simulink model "fourorder"  (R2023b)
settings: Solver=FixedStepAuto  StartTime=0.0  StopTime=100  FixedStep=0.001  RelTol=1e-3
values from neighbouring files (symbols this model uses):
  A = [-0.607110322581 0.050179746608 0 0 1 0 0 0.150121075269 -0.118469799623 0.253333333333 0 -1 ... (49 elements, 7x7)]    [data.mat]    (also in string1.m = [-(c1+cr)/J1 c1/J1 0 0 -k1/J1 0 0)
  AA = [-0.607110322581 0.050179746608 0 0 1 0 0 -1 0.150121075269 -0.118469799623 0.253333333333 0 ... (64 elements, 8x8)]    [data.mat]
  B = [0.0010752688172 0 0 0 0 0 0]    [data.mat]
  B2 = [0 0 0 -0.00211877963378 0 0 0 0.0010752688172 0 0 0 0 ... (14 elements, 7x2)]    [data.mat]    (also in demo_pid.m = -J \ [0; 1]; string1.m = [0 1/J1;0 0;0 0;-1/J4 0 ;0 0;0 0;0 0])
  BB = [0.0010752688172 0 0 0 0 0 0 0]    [data.mat]
  Bw = [0 0 0 -0.00211877963378 0 0 0 0]    [data.mat]
  C = [1 0 0 0 0 0 0]    [data.mat]    (also in string1.m = [1 0 0 0 0 0 0)
  C_3 = [1 0 0 0 0 0 0 0 0 0 0 1 ... (24 elements, 3x8)]    [data.mat]
  C_37 = [1 0 0 0 0 0 0 0 0 0 0 1 ... (21 elements, 3x7)]    [data.mat]
  G = [12.2186235804 178.38475641 -301.660194136 -80.857185539 -52.8926654988 -580.80827196 633.197555561]    [data.mat]
libraries: slpidlib x2, fuzblock x1
settings Model: Creator=ASUS  LastModifiedBy=86188
settings SolverCC: AlgebraicLoopSolver=TrustRegion
settings DebuggingCC: UnconnectedInputMsg=warning  UnconnectedOutputMsg=warning  UnconnectedLineMsg=warning
settings ModelReferenceCC: EnableRefExpFcnMdlSchedulingChecks=on
settings RTWCC: DLArmComputeVersion=19.05

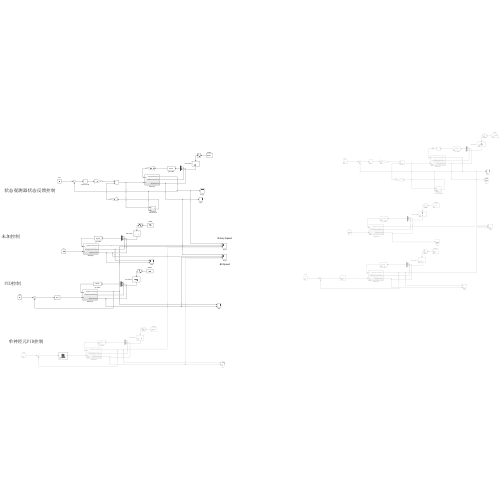
[thumbnail: Simulink's stored preview of the top-level diagram]
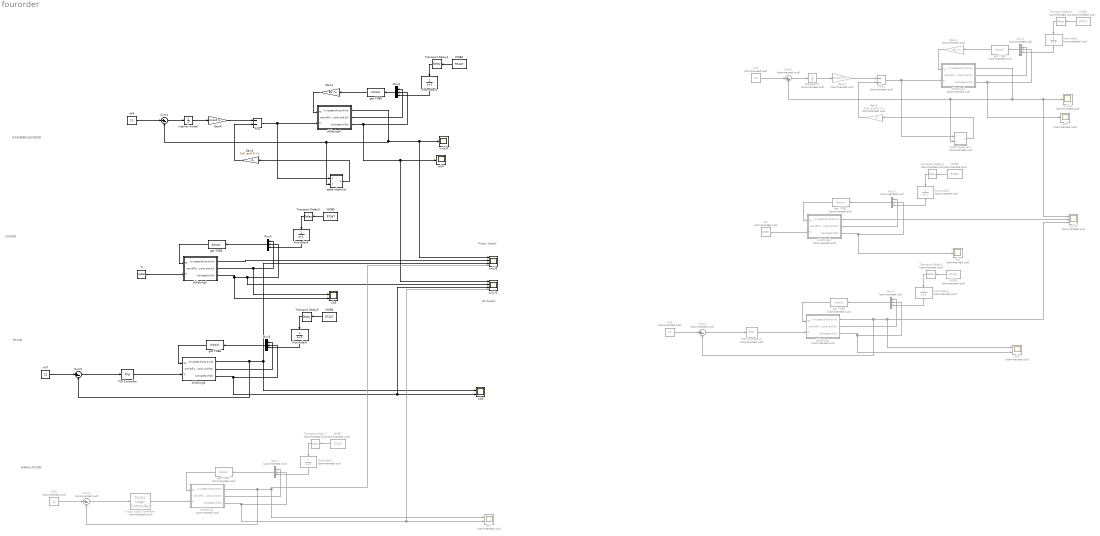
== system fourorder ==
  note: Rotary Speed
  note: 状态观测器状态反馈控制
  note: 未加控制
  note: PID控制
  note: Bit Speed
  note: 单神经元PID控制
  Fuzzy Logic Controller : fuzblock/Fuzzy Logic  Controller  Commented=on  FIS='drill.fis'  OutputSampleNumber=101  DataType=double  FuzzifiedInputs=off  RuleFiringStrengths=off  RuleOutputs=off  AggregatedOutputs=off  SimulateUsing=Interpreted execution  OutOfRangeInputValueMessage=warning  NoRuleFiredMessage=warning  EmptyOutputFuzzySetMessage=warning
  Gain1 : Gain  Commented=on  Gain=Bw  Multiplication=Matrix(K*u)
  Gain2 : Gain  Commented=on  Gain=Ks(1:end-1)  Multiplication=Matrix(K*u)
  Gain3 : Gain  Commented=on  Gain=Ks(end)  Multiplication=Matrix(K*u)
  Gain4 : Gain  Gain=Bw  Multiplication=Matrix(K*u)
  Gain5 : Gain  Gain=Ks(1:end-1)  Multiplication=Matrix(K*u)
  Gain6 : Gain  Gain=Ks(end)  Multiplication=Matrix(K*u)
  Integrator1 : Integrator  Commented=on
  Mux{1..3,7} (4 alike) : Mux  Commented=on  Inputs=3
  Mux4 : Mux  Inputs=3
  Mux5 : Mux  Inputs=3
  Mux6 : Mux  Inputs=3
  PID Controller : slpidlib/PID Controller  Controller=PI  Form=Parallel  TimeDomain=Continuous-time  UseExternalTs=off  SampleTime=-1  IntegratorMethod=Forward Euler  FilterMethod=Forward Euler  ControllerParametersSource=internal  P=1500  I=300  UseKiTs=off  D=0  N=100  UseFilter=on  TunerSelectOption=Transfer Function Based (PID Tuner App)  InitialConditionSource=internal  InitialConditionForIntegrator=0  InitialConditionForFilter=0  DifferentiatorICPrevScaledInput=0  ExternalReset=none  TrackingMode=off  Kt=1  LimitOutput=off  SatLimitsSource=internal  UpperSaturationLimit=inf  LowerSaturationLimit=-inf  LinearizeAsGain=on  AntiWindupMode=none  Kb=1  LimitIntegrator=off  UpperIntegratorSaturationLimit=inf  LowerIntegratorSaturationLimit=-inf  POutMin=[]  POutMax=[]  IOutMin=[]  IOutMax=[]  DOutMin=[]  DOutMax=[]  NOutMin=[]  NOutMax=[]  SumOutMin=[]  SumOutMax=[]  SaturationOutMin=[]  SaturationOutMax=[]  PParamMin=[]  PParamMax=[]  IParamMin=[]  IParamMax=[]  DParamMin=[]  DParamMax=[]  NParamMin=[]  NParamMax=[]  KbParamMin=[]  KbParamMax=[]  KtParamMin=[]  KtParamMax=[]  KbOutMin=[]  KbOutMax=[]  KtOutMin=[]  KtOutMax=[]  IntegratorOutMin=[]  IntegratorOutMax=[]  FilterOutMin=[]  FilterOutMax=[]  SumI1OutMin=[]  SumI1OutMax=[]  SumI2OutMin=[]  SumI2OutMax=[]  SumI3OutMin=[]  SumI3OutMax=[]  SumI4OutMin=[]  SumI4OutMax=[]  SumDOutMin=[]  SumDOutMax=[]  DifferentiatorOutMin=[]  DifferentiatorOutMax=[]  FilterDiffOutCoefMin=[]  FilterDiffOutCoefMax=[]  ReciprocalOutMin=[]  ReciprocalOutMax=[]  SumDenOutMin=[]  SumDenOutMax=[]  SumNumOutMin=[]  SumNumOutMax=[]  DivideOutMin=[]  DivideOutMax=[]  UdiffTsProdOutMin=[]  UdiffTsProdOutMax=[]  NTsProdOutMin=[]  NTsProdOutMax=[]  UintegralTsProdOutMin=[]  UintegralTsProdOutMax=[]  UngainTsProdOutMin=[]  UngainTsProdOutMax=[]  ClampingZeroOutDataTypeStr=Inherit: Inherit via back propagation  ClampingZeroOutMin=[]  ClampingZeroOutMax=[]  FilterDenConstantOutDataTypeStr=Inherit: Inherit via back propagation  FilterDenConstantOutMin=[]  FilterDenConstantOutMax=[]  PCopyOutDataTypeStr=Inherit: Inherit via back propagation  PCopyOutMin=[]  PCopyOutMax=[]  NCopyOutDataTypeStr=Inherit: Inherit via back propagation  NCopyOutMin=[]  NCopyOutMax=[]  IntegratorContinuousStateAttributes=''  IntegratorStateMustResolveToSignalObject=off  IntegratorRTWStateStorageClass=Auto  FilterContinuousStateAttributes=''  FilterStateMustResolveToSignalObject=off  FilterRTWStateStorageClass=Auto  ParallelPVariant=InternalParameters  IdealPVariant=Disabled  IVariant=InternalParameters  DVariant=Disabled  IntegratorVariant=Continuous  SatVariant=Disabled  AWVariant=Passthrough  PCopyVariant=Disabled  TRVariant=Disabled  FdbkBlocksVariant=Forward  IdealPFdbkVariant=Disabled  SatFdbkVariant=Disabled  DerivativeFilterVariant=Disabled  NVariant=Disabled  NCopyVariant=Disabled_SignalSpec  FilterICVariant=Disabled  IntegratorICVariant=InternalICs  ExternalResetVariant=Disabled  TRSumVariant=Passthrough  SumFdbkVariant=Disabled  SumVariant=Sum_PI  TsampFilterVariant=InternalTs  TsampNgainVariant=Passthrough  TsampIntegralVariant=Disabled_SignalSpec  ExternalSaturationOutDataTypeStr=Inherit: Same as second input
  PID Controller1 : slpidlib/PID Controller  Commented=on  Controller=PI  Form=Parallel  TimeDomain=Continuous-time  UseExternalTs=off  SampleTime=-1  IntegratorMethod=Forward Euler  FilterMethod=Forward Euler  ControllerParametersSource=internal  P=1000  I=100  UseKiTs=off  D=0  N=100  UseFilter=on  TunerSelectOption=Transfer Function Based (PID Tuner App)  InitialConditionSource=internal  InitialConditionForIntegrator=0  InitialConditionForFilter=0  DifferentiatorICPrevScaledInput=0  ExternalReset=none  TrackingMode=off  Kt=1  LimitOutput=off  SatLimitsSource=internal  UpperSaturationLimit=inf  LowerSaturationLimit=-inf  LinearizeAsGain=on  AntiWindupMode=none  Kb=1  LimitIntegrator=off  UpperIntegratorSaturationLimit=inf  LowerIntegratorSaturationLimit=-inf  POutMin=[]  POutMax=[]  IOutMin=[]  IOutMax=[]  DOutMin=[]  DOutMax=[]  NOutMin=[]  NOutMax=[]  SumOutMin=[]  SumOutMax=[]  SaturationOutMin=[]  SaturationOutMax=[]  PParamMin=[]  PParamMax=[]  IParamMin=[]  IParamMax=[]  DParamMin=[]  DParamMax=[]  NParamMin=[]  NParamMax=[]  KbParamMin=[]  KbParamMax=[]  KtParamMin=[]  KtParamMax=[]  KbOutMin=[]  KbOutMax=[]  KtOutMin=[]  KtOutMax=[]  IntegratorOutMin=[]  IntegratorOutMax=[]  FilterOutMin=[]  FilterOutMax=[]  SumI1OutMin=[]  SumI1OutMax=[]  SumI2OutMin=[]  SumI2OutMax=[]  SumI3OutMin=[]  SumI3OutMax=[]  SumI4OutMin=[]  SumI4OutMax=[]  SumDOutMin=[]  SumDOutMax=[]  DifferentiatorOutMin=[]  DifferentiatorOutMax=[]  FilterDiffOutCoefMin=[]  FilterDiffOutCoefMax=[]  ReciprocalOutMin=[]  ReciprocalOutMax=[]  SumDenOutMin=[]  SumDenOutMax=[]  SumNumOutMin=[]  SumNumOutMax=[]  DivideOutMin=[]  DivideOutMax=[]  UdiffTsProdOutMin=[]  UdiffTsProdOutMax=[]  NTsProdOutMin=[]  NTsProdOutMax=[]  UintegralTsProdOutMin=[]  UintegralTsProdOutMax=[]  UngainTsProdOutMin=[]  UngainTsProdOutMax=[]  ClampingZeroOutDataTypeStr=Inherit: Inherit via back propagation  ClampingZeroOutMin=[]  ClampingZeroOutMax=[]  FilterDenConstantOutDataTypeStr=Inherit: Inherit via back propagation  FilterDenConstantOutMin=[]  FilterDenConstantOutMax=[]  PCopyOutDataTypeStr=Inherit: Inherit via back propagation  PCopyOutMin=[]  PCopyOutMax=[]  NCopyOutDataTypeStr=Inherit: Inherit via back propagation  NCopyOutMin=[]  NCopyOutMax=[]  IntegratorContinuousStateAttributes=''  IntegratorStateMustResolveToSignalObject=off  IntegratorRTWStateStorageClass=Auto  FilterContinuousStateAttributes=''  FilterStateMustResolveToSignalObject=off  FilterRTWStateStorageClass=Auto  ParallelPVariant=InternalParameters  IdealPVariant=Disabled  IVariant=InternalParameters  DVariant=Disabled  IntegratorVariant=Continuous  SatVariant=Disabled  AWVariant=Passthrough  PCopyVariant=Disabled  TRVariant=Disabled  FdbkBlocksVariant=Forward  IdealPFdbkVariant=Disabled  SatFdbkVariant=Disabled  DerivativeFilterVariant=Disabled  NVariant=Disabled  NCopyVariant=Disabled_SignalSpec  FilterICVariant=Disabled  IntegratorICVariant=InternalICs  ExternalResetVariant=Disabled  TRSumVariant=Passthrough  SumFdbkVariant=Disabled  SumVariant=Sum_PI  TsampFilterVariant=InternalTs  TsampNgainVariant=Passthrough  TsampIntegralVariant=Disabled_SignalSpec  ExternalSaturationOutDataTypeStr=Inherit: Same as second input
  Plus : Sum  Inputs=--
  Plus1 : Sum  Commented=on  Inputs=--
  Sum1 : Sum  Commented=on  Inputs=|+-
  Sum2 : Sum  Commented=on  Inputs=|+-
  Sum3 : Sum  Commented=on  Inputs=|+-
  Sum4 : Sum  Inputs=|+-
  Sum5 : Sum  Inputs=|+-
  Tr : Constant  Value=10000
  Tr1 : Constant  Commented=on  Value=10000
  Transport Delay{1..3,7} (4 alike) : TransportDelay  Commented=on  DelayTime=50  InitialOutput=100000
  Transport Delay4 : TransportDelay  DelayTime=50  InitialOutput=100000
  Transport Delay5 : TransportDelay  DelayTime=50  InitialOutput=100000
  Transport Delay6 : TransportDelay  DelayTime=50  InitialOutput=100000
  WOB{1..3,7} (4 alike) : Constant  Commented=on  Value=97347
  WOB4 : Constant  Value=97347
  WOB5 : Constant  Value=97347
  WOB6 : Constant  Value=97347
  drillstring1 : Subsystem  Commented=on
  drillstring2 : Subsystem  Commented=on
  drillstring3 : Subsystem  Commented=on
  drillstring4 : Subsystem
  drillstring5 : Subsystem
  drillstring6 : Subsystem
  drillstring7 : Subsystem  Commented=on
  first-order{1..3,7} (4 alike) : TransferFcn  Commented=on  Denominator=[1 1]
  first-order4 : TransferFcn  Denominator=[1 1]
  first-order5 : TransferFcn  Denominator=[1 1]
  first-order6 : TransferFcn  Denominator=[1 1]
  get TOB{1..3,7} (4 alike) : S-Function  Commented=on  FunctionName=bitrock  SFunctionDeploymentMode=off  EnableBusSupport=off
  get TOB4 : S-Function  FunctionName=bitrock  SFunctionDeploymentMode=off  EnableBusSupport=off
  get TOB5 : S-Function  FunctionName=bitrock  SFunctionDeploymentMode=off  EnableBusSupport=off
  get TOB6 : S-Function  FunctionName=bitrock  SFunctionDeploymentMode=off  EnableBusSupport=off
  internal model : Integrator
  r(t)1 : Constant  Commented=on  Value=12
  r(t)2 : Constant  Commented=on  Value=12
  r(t)3 : Constant  Commented=on  Value=12
  r(t)4 : Constant  Value=12
  r(t)7 : Constant  Value=12
  state observer : Subsystem
  state observer1 : Subsystem  Commented=on
  wb1 : Scope  Commented=on
  wb2 : Scope  Commented=on
  wb3 : Scope  Commented=on  NumInputPorts=2
  wb4 : Scope
  wb5 : Scope  NumInputPorts=2
  wb6 : Scope  NumInputPorts=2
  wb7 : Scope  Commented=on  NumInputPorts=2
  wr(y)1 : Scope  Commented=on
  wr(y)2 : Scope  Commented=on  NumInputPorts=3
  wr(y)3 : Scope  NumInputPorts=4
  wr(y)4 : Scope
  wr(y)5 : Scope  NumInputPorts=4
  wires:
  state observer/1(Out1) -> Gain5/1
  first-order4/1 -> Mux4/3
  Transport Delay4/1 -> first-order4/1
  drillstring4/3(wb(speed of bit)) -> wr(y)3/1, wb4/1, Mux4/2
  Mux4/1 -> get TOB4/1
  drillstring4/2(wer(diff of collar and bit)) -> Mux4/1
  drillstring4/1(wr(speed of top drive)) -> Sum4/2, state observer/2(In2), wr(y)5/1, wr(y)4/1
  r(t)4/1 -> Sum4/1
  Sum4/1 -> internal model/1
  WOB4/1 -> Transport Delay4/1
  get TOB4/1 -> Gain4/1
  Plus/1 -> drillstring4/2(Tr), state observer/1(In1)
  Gain5/1 -> Plus/2
  Gain6/1 -> Plus/1
  internal model/1 -> Gain6/1
  Gain4/1 -> drillstring4/1(Tb)
  drillstring5/1(wr(speed of top drive)) -> wr(y)5/2
  WOB5/1 -> Transport Delay5/1
  drillstring5/2(wer(diff of collar and bit)) -> wb5/1, Mux5/1
  first-order5/1 -> Mux5/3
  Mux5/1 -> get TOB5/1
  drillstring5/3(wb(speed of bit)) -> wb5/2, wr(y)3/2, Mux5/2
  get TOB5/1 -> drillstring5/1(Tb)
  Transport Delay5/1 -> first-order5/1
  Tr/1 -> drillstring5/2(Tr)
  Sum5/1 -> PID Controller/1
  drillstring6/2(wer(diff of collar and bit)) -> Mux6/1
  Mux6/1 -> get TOB6/1
  Transport Delay6/1 -> first-order6/1
  get TOB6/1 -> drillstring6/1(Tb)
  first-order6/1 -> Mux6/3
  drillstring6/3(wb(speed of bit)) -> wr(y)3/3, wb6/2, Mux6/2
  WOB6/1 -> Transport Delay6/1
  drillstring6/1(wr(speed of top drive)) -> Sum5/2, wb6/1, wr(y)5/3
  r(t)7/1 -> Sum5/1
  PID Controller/1 -> drillstring6/2(Tr)
  Plus1/1 -> drillstring1/2(Tr), state observer1/1(In1)
  drillstring2/1(wr(speed of top drive)) -> wr(y)2/2
  drillstring3/3(wb(speed of bit)) -> wb3/2, Mux3/2
  PID Controller1/1 -> drillstring3/2(Tr)
  first-order3/1 -> Mux3/3
  WOB3/1 -> Transport Delay3/1
  drillstring3/2(wer(diff of collar and bit)) -> Mux3/1
  Mux3/1 -> get TOB3/1
  r(t)2/1 -> Sum2/1
  Gain2/1 -> Plus1/2
  Gain3/1 -> Plus1/1
  Transport Delay3/1 -> first-order3/1
  Integrator1/1 -> Gain3/1
  get TOB3/1 -> drillstring3/1(Tb)
  drillstring2/2(wer(diff of collar and bit)) -> Mux2/1
  Mux2/1 -> get TOB2/1
  Transport Delay2/1 -> first-order2/1
  get TOB2/1 -> drillstring2/1(Tb)
  first-order2/1 -> Mux2/3
  get TOB1/1 -> Gain1/1
  WOB2/1 -> Transport Delay2/1
  Sum2/1 -> PID Controller1/1
  Sum1/1 -> Integrator1/1
  drillstring1/1(wr(speed of top drive)) -> Sum1/2, state observer1/2(In2), wr(y)2/1, wr(y)1/1
  WOB1/1 -> Transport Delay1/1
  r(t)1/1 -> Sum1/1
  drillstring1/2(wer(diff of collar and bit)) -> Mux1/1
  first-order1/1 -> Mux1/3
  Tr1/1 -> drillstring2/2(Tr)
  drillstring3/1(wr(speed of top drive)) -> Sum2/2, wb3/1, wr(y)2/3
  drillstring2/3(wb(speed of bit)) -> wb2/1, Mux2/2
  Mux1/1 -> get TOB1/1
  drillstring1/3(wb(speed of bit)) -> wb1/1, Mux1/2
  Gain1/1 -> drillstring1/1(Tb)
  state observer1/1(Out1) -> Gain2/1
  Transport Delay1/1 -> first-order1/1
  drillstring7/1(wr(speed of top drive)) -> Sum3/2, wr(y)5/4, wb7/1
  Fuzzy Logic Controller/1 -> drillstring7/2(Tr)
  drillstring7/3(wb(speed of bit)) -> wr(y)3/4, wb7/2, Mux7/2
  Transport Delay7/1 -> first-order7/1
  WOB7/1 -> Transport Delay7/1
  get TOB7/1 -> drillstring7/1(Tb)
  drillstring7/2(wer(diff of collar and bit)) -> Mux7/1
  first-order7/1 -> Mux7/3
  Sum3/1 -> Fuzzy Logic Controller/1
  r(t)3/1 -> Sum3/1
  Mux7/1 -> get TOB7/1

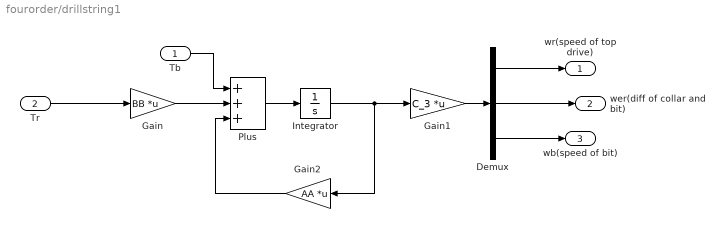
== system fourorder/drillstring1 ==
  Tb : Inport
  Tr : Inport  Port=2
  Demux : Demux  Outputs=3
  Gain : Gain  Gain=BB  Multiplication=Matrix(K*u)
  Gain1 : Gain  Gain=C_3  Multiplication=Matrix(K*u)
  Gain2 : Gain  Gain=AA  Multiplication=Matrix(K*u)
  Integrator : Integrator
  Plus : Sum  Inputs=+++
  wr(speed of top drive) : Outport
  wer(diff of collar and bit) : Outport  Port=2
  wb(speed of bit) : Outport  Port=3
  wires:
  Demux/3 -> wb(speed of bit)/1
  Integrator/1 -> Gain2/1, Gain1/1
  Plus/1 -> Integrator/1
  Tr/1 -> Gain/1
  Demux/1 -> wr(speed of top drive)/1
  Gain2/1 -> Plus/3
  Gain1/1 -> Demux/1
  Demux/2 -> wer(diff of collar and bit)/1
  Tb/1 -> Plus/1
  Gain/1 -> Plus/2

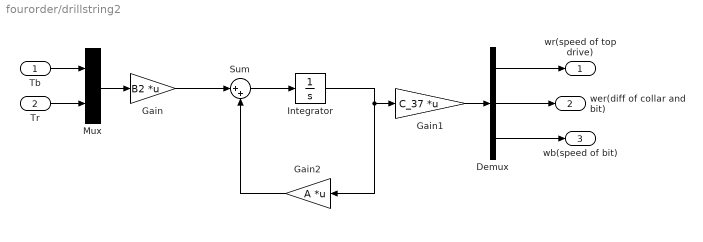
== system fourorder/drillstring2 ==
  Tb : Inport
  Tr : Inport  Port=2
  Demux : Demux  Outputs=3
  Gain : Gain  Gain=B2  Multiplication=Matrix(K*u)
  Gain1 : Gain  Gain=C_37  Multiplication=Matrix(K*u)
  Gain2 : Gain  Gain=A  Multiplication=Matrix(K*u)
  Integrator : Integrator
  Mux : Mux  Inputs=2
  Sum : Sum  Inputs=|++
  wr(speed of top drive) : Outport
  wer(diff of collar and bit) : Outport  Port=2
  wb(speed of bit) : Outport  Port=3
  wires:
  Demux/3 -> wb(speed of bit)/1
  Integrator/1 -> Gain2/1, Gain1/1
  Sum/1 -> Integrator/1
  Tr/1 -> Mux/2
  Demux/1 -> wr(speed of top drive)/1
  Gain2/1 -> Sum/2
  Gain1/1 -> Demux/1
  Demux/2 -> wer(diff of collar and bit)/1
  Tb/1 -> Mux/1
  Gain/1 -> Sum/1
  Mux/1 -> Gain/1

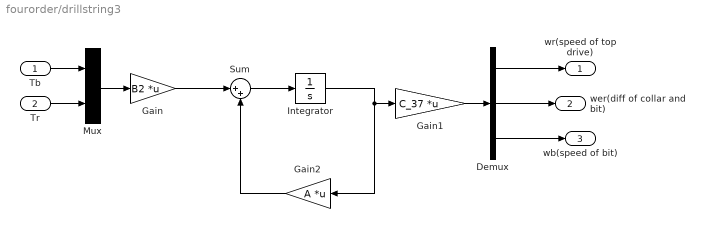
== system fourorder/drillstring3 ==
  Tb : Inport
  Tr : Inport  Port=2
  Demux : Demux  Outputs=3
  Gain : Gain  Gain=B2  Multiplication=Matrix(K*u)
  Gain1 : Gain  Gain=C_37  Multiplication=Matrix(K*u)
  Gain2 : Gain  Gain=A  Multiplication=Matrix(K*u)
  Integrator : Integrator
  Mux : Mux  Inputs=2
  Sum : Sum  Inputs=|++
  wr(speed of top drive) : Outport
  wer(diff of collar and bit) : Outport  Port=2
  wb(speed of bit) : Outport  Port=3
  wires:
  Demux/3 -> wb(speed of bit)/1
  Integrator/1 -> Gain2/1, Gain1/1
  Sum/1 -> Integrator/1
  Tr/1 -> Mux/2
  Demux/1 -> wr(speed of top drive)/1
  Gain2/1 -> Sum/2
  Gain1/1 -> Demux/1
  Demux/2 -> wer(diff of collar and bit)/1
  Tb/1 -> Mux/1
  Gain/1 -> Sum/1
  Mux/1 -> Gain/1

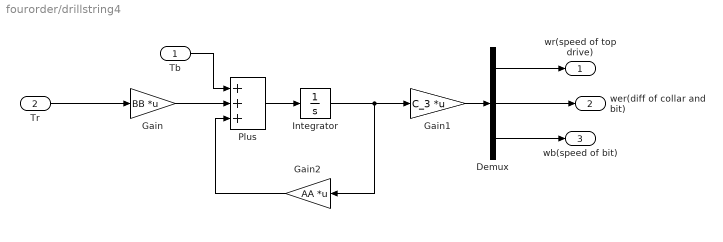
== system fourorder/drillstring4 ==
  Tb : Inport
  Tr : Inport  Port=2
  Demux : Demux  Outputs=3
  Gain : Gain  Gain=BB  Multiplication=Matrix(K*u)
  Gain1 : Gain  Gain=C_3  Multiplication=Matrix(K*u)
  Gain2 : Gain  Gain=AA  Multiplication=Matrix(K*u)
  Integrator : Integrator
  Plus : Sum  Inputs=+++
  wr(speed of top drive) : Outport
  wer(diff of collar and bit) : Outport  Port=2
  wb(speed of bit) : Outport  Port=3
  wires:
  Demux/3 -> wb(speed of bit)/1
  Integrator/1 -> Gain2/1, Gain1/1
  Plus/1 -> Integrator/1
  Tr/1 -> Gain/1
  Demux/1 -> wr(speed of top drive)/1
  Gain2/1 -> Plus/3
  Gain1/1 -> Demux/1
  Demux/2 -> wer(diff of collar and bit)/1
  Tb/1 -> Plus/1
  Gain/1 -> Plus/2

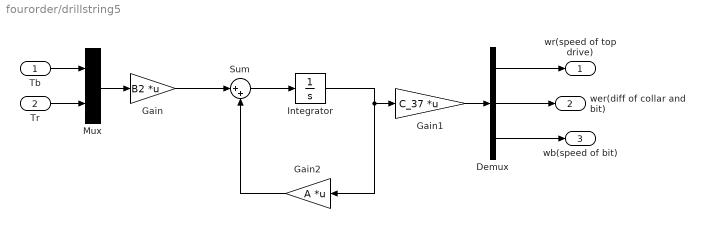
== system fourorder/drillstring5 ==
  Tb : Inport
  Tr : Inport  Port=2
  Demux : Demux  Outputs=3
  Gain : Gain  Gain=B2  Multiplication=Matrix(K*u)
  Gain1 : Gain  Gain=C_37  Multiplication=Matrix(K*u)
  Gain2 : Gain  Gain=A  Multiplication=Matrix(K*u)
  Integrator : Integrator
  Mux : Mux  Inputs=2
  Sum : Sum  Inputs=|++
  wr(speed of top drive) : Outport
  wer(diff of collar and bit) : Outport  Port=2
  wb(speed of bit) : Outport  Port=3
  wires:
  Demux/3 -> wb(speed of bit)/1
  Integrator/1 -> Gain2/1, Gain1/1
  Sum/1 -> Integrator/1
  Tr/1 -> Mux/2
  Demux/1 -> wr(speed of top drive)/1
  Gain2/1 -> Sum/2
  Gain1/1 -> Demux/1
  Demux/2 -> wer(diff of collar and bit)/1
  Tb/1 -> Mux/1
  Gain/1 -> Sum/1
  Mux/1 -> Gain/1

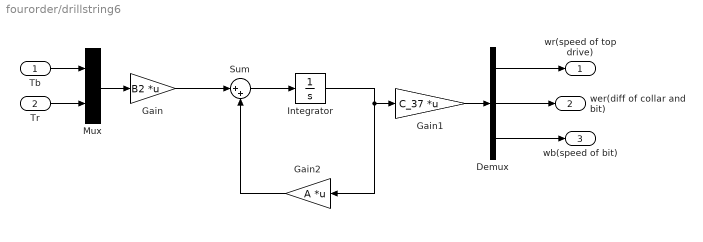
== system fourorder/drillstring6 ==
  Tb : Inport
  Tr : Inport  Port=2
  Demux : Demux  Outputs=3
  Gain : Gain  Gain=B2  Multiplication=Matrix(K*u)
  Gain1 : Gain  Gain=C_37  Multiplication=Matrix(K*u)
  Gain2 : Gain  Gain=A  Multiplication=Matrix(K*u)
  Integrator : Integrator
  Mux : Mux  Inputs=2
  Sum : Sum  Inputs=|++
  wr(speed of top drive) : Outport
  wer(diff of collar and bit) : Outport  Port=2
  wb(speed of bit) : Outport  Port=3
  wires:
  Demux/3 -> wb(speed of bit)/1
  Integrator/1 -> Gain2/1, Gain1/1
  Sum/1 -> Integrator/1
  Tr/1 -> Mux/2
  Demux/1 -> wr(speed of top drive)/1
  Gain2/1 -> Sum/2
  Gain1/1 -> Demux/1
  Demux/2 -> wer(diff of collar and bit)/1
  Tb/1 -> Mux/1
  Gain/1 -> Sum/1
  Mux/1 -> Gain/1

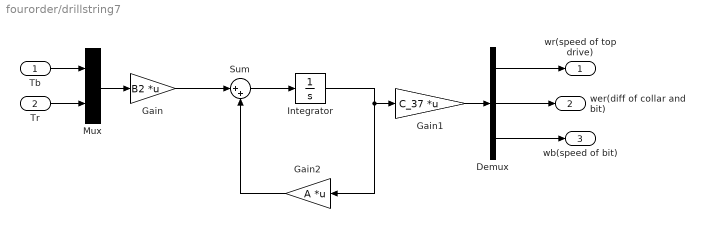
== system fourorder/drillstring7 ==
  Tb : Inport
  Tr : Inport  Port=2
  Demux : Demux  Outputs=3
  Gain : Gain  Gain=B2  Multiplication=Matrix(K*u)
  Gain1 : Gain  Gain=C_37  Multiplication=Matrix(K*u)
  Gain2 : Gain  Gain=A  Multiplication=Matrix(K*u)
  Integrator : Integrator
  Mux : Mux  Inputs=2
  Sum : Sum  Inputs=|++
  wr(speed of top drive) : Outport
  wer(diff of collar and bit) : Outport  Port=2
  wb(speed of bit) : Outport  Port=3
  wires:
  Demux/3 -> wb(speed of bit)/1
  Integrator/1 -> Gain2/1, Gain1/1
  Sum/1 -> Integrator/1
  Tr/1 -> Mux/2
  Demux/1 -> wr(speed of top drive)/1
  Gain2/1 -> Sum/2
  Gain1/1 -> Demux/1
  Demux/2 -> wer(diff of collar and bit)/1
  Tb/1 -> Mux/1
  Gain/1 -> Sum/1
  Mux/1 -> Gain/1

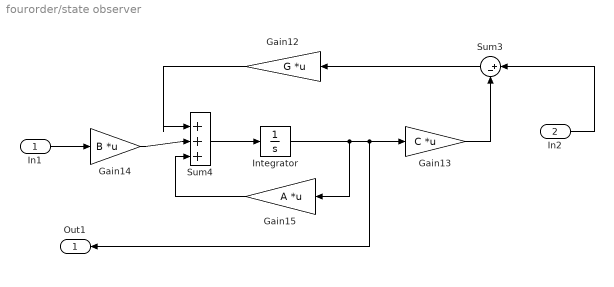
== system fourorder/state observer ==
  In1 : Inport
  In2 : Inport  Port=2
  Gain12 : Gain  Gain=G  Multiplication=Matrix(K*u)
  Gain13 : Gain  Gain=C  Multiplication=Matrix(K*u)
  Gain14 : Gain  Gain=B  Multiplication=Matrix(K*u)
  Gain15 : Gain  Gain=A  Multiplication=Matrix(K*u)
  Integrator : Integrator
  Sum3 : Sum  Inputs=|+-
  Sum4 : Sum  Inputs=|+++
  Out1 : Outport
  wires:
  Sum3/1 -> Gain12/1
  Gain13/1 -> Sum3/2
  Gain14/1 -> Sum4/2
  Sum4/1 -> Integrator/1
  Gain15/1 -> Sum4/3
  Gain12/1 -> Sum4/1
  In2/1 -> Sum3/1
  Integrator/1 -> Out1/1, Gain13/1, Gain15/1
  In1/1 -> Gain14/1

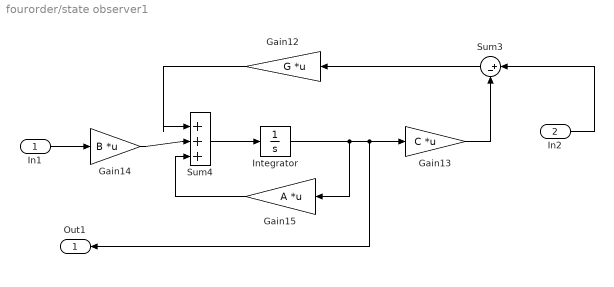
== system fourorder/state observer1 ==
  In1 : Inport
  In2 : Inport  Port=2
  Gain12 : Gain  Gain=G  Multiplication=Matrix(K*u)
  Gain13 : Gain  Gain=C  Multiplication=Matrix(K*u)
  Gain14 : Gain  Gain=B  Multiplication=Matrix(K*u)
  Gain15 : Gain  Gain=A  Multiplication=Matrix(K*u)
  Integrator : Integrator
  Sum3 : Sum  Inputs=|+-
  Sum4 : Sum  Inputs=|+++
  Out1 : Outport
  wires:
  Sum3/1 -> Gain12/1
  Gain13/1 -> Sum3/2
  Gain14/1 -> Sum4/2
  Sum4/1 -> Integrator/1
  Gain15/1 -> Sum4/3
  Gain12/1 -> Sum4/1
  In2/1 -> Sum3/1
  Integrator/1 -> Out1/1, Gain13/1, Gain15/1
  In1/1 -> Gain14/1
